simulink model "arduino_control_loop"  (R2024a)
settings: Solver=VariableStepAuto  StartTime=0.0  StopTime=10000.0  RelTol=1e-3
values from neighbouring files (symbols this model uses):
  A_air = 0.00588710854841    [run1.mat]    (also in run2.mat)
  Cs = 0.9    [run1.mat]    (also in run2.mat)
  D_offset = 0.220382951982    [run1.mat]    (also in run2.mat)
  h = 0.0127000254001    [run1.mat]    (also in run2.mat)
  K = 0.0866241164464    [run1.mat]    (also in run2.mat)
  m = 100    [run1.mat]    (also in run2.mat)
  T_f = 21    [run1.mat]    (also in run2.mat)
settings Model: Creator=veswaranandam  LastModifiedBy=veswaranandam

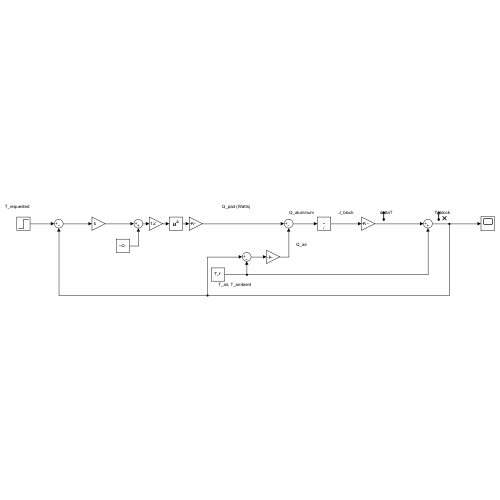
[thumbnail: Simulink's stored preview of the top-level diagram]
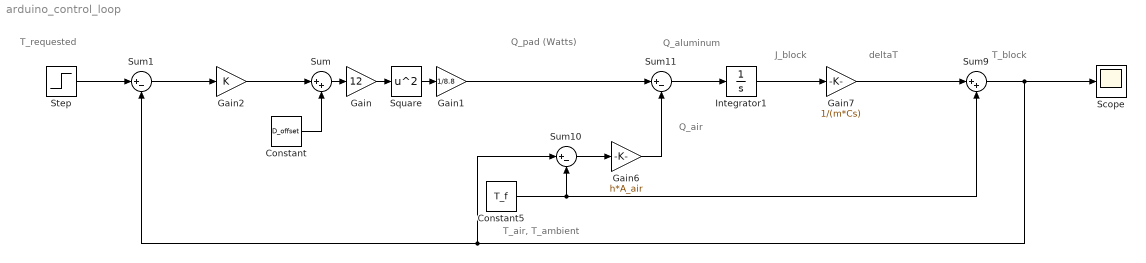
== system arduino_control_loop ==
  note: T_requested
  note: deltaT
  note: Q_aluminum
  note: Q_pad (Watts)
  note: J_block
  note: T_block
  note: Q_air
  note: T_air, T_ambient
  Constant : Constant  Value=D_offset
  Constant5 : Constant  Value=T_f
  Gain : Gain  Gain=12
  Gain1 : Gain  Gain=1/8.8
  Gain2 : Gain  Gain=K
  Gain6 : Gain  Gain=h*A_air
  Gain7 : Gain  Gain=1/(m*Cs)
  Integrator1 : Integrator
  Scope : Scope
  Square : Math  Operator=square
  Step : Step  Before=25  After=29  SampleTime=0
  Sum : Sum  Inputs=|++
  Sum1 : Sum  Inputs=|+-
  Sum10 : Sum  Inputs=|+-
  Sum11 : Sum  Inputs=|+-
  Sum9 : Sum  Inputs=|++
  wires:
  Sum9/1 -> Scope/1, Sum1/2, Sum10/1
  Sum11/1 -> Integrator1/1
  Gain7/1 -> Sum9/1
  Gain6/1 -> Sum11/2
  Constant5/1 -> Sum9/2, Sum10/2
  Sum10/1 -> Gain6/1
  Gain1/1 -> Sum11/1
  Integrator1/1 -> Gain7/1
  Gain/1 -> Square/1
  Square/1 -> Gain1/1
  Sum/1 -> Gain/1
  Constant/1 -> Sum/2
  Gain2/1 -> Sum/1
  Step/1 -> Sum1/1
  Sum1/1 -> Gain2/1
